simulink model "DCDC3_ZCL"  (R2024a)
settings: Solver=FixedStepDiscrete  StartTime=0.0  StopTime=Tsim_outLoop  FixedStep=Tsw  RelTol=1e-3
undefined symbols (not defined in the file): deadtimesw, ILmax, kaw_i, kaw_v, ki_i, ki_v, kp_i, kp_v, Rload, Tstep, Tsw, VinNom, VLlim, VoutNom, zden_aaf, zden_Integrator, zden_plant_i, zden_plant_v, znum_aaf, znum_Integrator, znum_plant_i, znum_plant_v
libraries: simulink x10, spsTriangleGeneratorLib x6
settings Model: Creator=nicholas  LastModifiedBy=nicholas
settings RTWCC: GPUComputeCapability=3.5

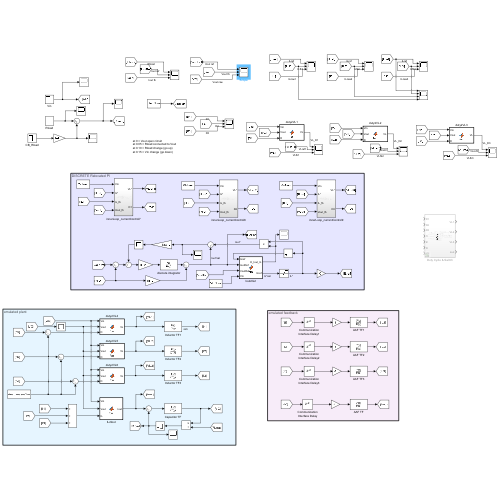
[thumbnail: Simulink's stored preview of the top-level diagram]
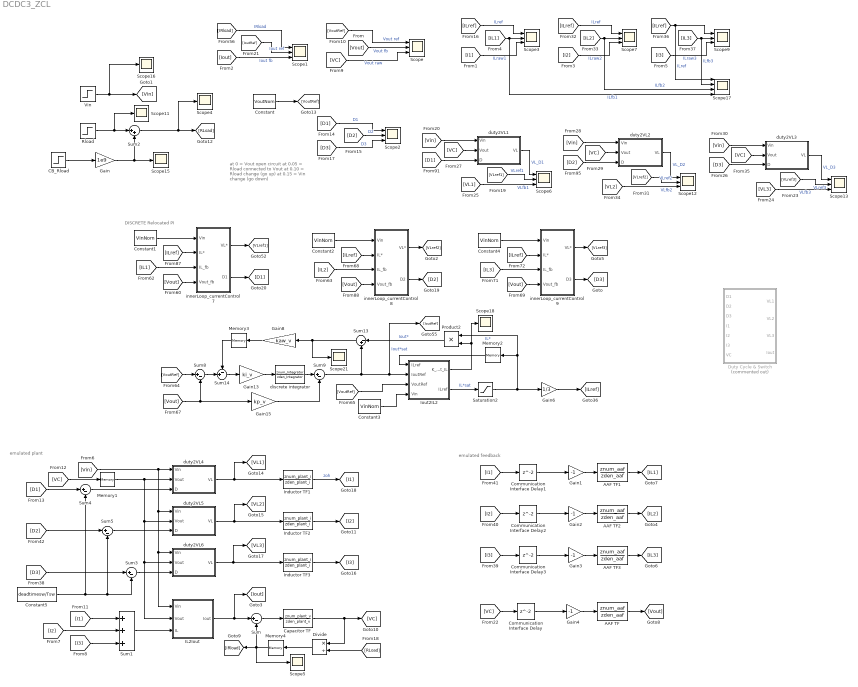
== system DCDC3_ZCL ==
  note: emulated plant
  note: emulated feedback
  note: DISCRETE Relocated PI
  note: at 0 = Vout open circuit
      | at 0.05 = Rload connected to Vout
      | at 0.10 = Rload change (go up)
      | at 0.15 = Vin change (go down)
  AAF TF{,1..3} (4 alike) : DiscreteTransferFcn  Numerator=znum_aaf  Denominator=zden_aaf
  CB_Rload : Step  Time=0.05  Before=1  After=0  SampleTime=0
  Capacitor TF : DiscreteTransferFcn  Numerator=znum_plant_v  Denominator=zden_plant_v
  Communication Interface Delay{,1..3} (4 alike) : Delay
  Constant : Constant  Value=VoutNom
  Constant{1..4} (4 alike) : Constant  Value=VinNom
  Constant5 : Constant  Value=deadtimesw/Tsw
  Divide : Product  Inputs=*/
  Duty Cycle & Switch : Subsystem  Commented=on
  Gain : Gain  Gain=1e9
  Gain{1..4} (4 alike) : Gain  Gain=-1
  Gain13 : Gain  Gain=ki_v
  Gain15 : Gain  Gain=kp_v
  Gain6 : Gain  Gain=1/3
  Gain8 : Gain  Gain=kaw_v
  IL2Iout : MATLAB Function  TreatAsAtomicUnit=on
  Inductor TF1 : DiscreteTransferFcn  Numerator=znum_plant_i  Denominator=zden_plant_i
  Inductor TF2 : DiscreteTransferFcn  Numerator=znum_plant_i  Denominator=zden_plant_i
  Inductor TF3 : DiscreteTransferFcn  Numerator=znum_plant_i  Denominator=zden_plant_i
  Iout2IL2 : MATLAB Function  TreatAsAtomicUnit=on
  Memory{1..4} (4 alike) : Memory  InheritSampleTime=on
  Product2 : Product
  Rload : Step  Time=0.10  Before=Rload  After=Rload*2  SampleTime=0
  Saturation2 : Saturate  UpperLimit=ILmax  LowerLimit=-ILmax
  Scope{,1..3,6..7,9,12..13} (9 alike) : Scope  NumInputPorts=3
  Scope{4..5,11,15..16,18,21} (7 alike) : Scope
  Scope17 : Scope  NumInputPorts=4
  Sum{,3..5,8..9} (6 alike) : Sum  Inputs=|+-
  Sum1 : Sum  Inputs=+++
  Sum13 : Sum  Inputs=|-+
  Sum14 : Sum  Inputs=-+|
  Sum2 : Sum  Inputs=|++
  Vin : Step  Time=0.15  Before=VinNom  After=20  SampleTime=0
  discrete integrator : DiscreteTransferFcn  Numerator=znum_Integrator  Denominator=zden_Integrator
  duty2VL1 : MATLAB Function  TreatAsAtomicUnit=on
  duty2VL2 : MATLAB Function  TreatAsAtomicUnit=on
  duty2VL3 : MATLAB Function  TreatAsAtomicUnit=on
  duty2VL4 : MATLAB Function  TreatAsAtomicUnit=on
  duty2VL5 : MATLAB Function  TreatAsAtomicUnit=on
  duty2VL6 : MATLAB Function  TreatAsAtomicUnit=on
  innerLoop_currentControl7 : Subsystem
  innerLoop_currentControl8 : Subsystem
  innerLoop_currentControl9 : Subsystem
  wires:
  [Iout] -> Scope1/3  "Iout fb"
  [Vout] -> Scope/2  "Vout fb"
  [IL1] -> Scope17/4, Scope3/2  "ILfb1"
  [ILref] -> Scope3/1  "ILref"
  [VoutRef] -> Scope/1  "Vout ref"
  [IoutRef] -> Scope1/2  "Iout ref"
  Constant/1 -> [VoutRef]
  [IL2] -> Scope7/2, Scope17/3  "ILfb2"
  [ILref] -> Scope7/1  "ILref"
  [IL3] -> Scope17/2, Scope9/2  "ILfb3"
  [ILref] -> Scope17/1, Scope9/1  "ILref"
  [IRload] -> Scope1/1  "IRload"
  [I1] -> Scope3/3  "ILraw1"
  [I2] -> Scope7/3  "ILraw2"
  [I3] -> Scope9/3  "ILraw3"
  Saturation2/1 -> Product2/1, Memory2/1, Gain6/1  "IL*"
  [IL1] -> innerLoop_currentControl7/3(IL_fb)
  [Vout] -> innerLoop_currentControl8/4(Vout_fb)
  Constant4/1 -> innerLoop_currentControl9/1(Vin)
  Gain13/1 -> discrete integrator/1
  [VoutRef] -> Sum8/1
  [Vout] -> innerLoop_currentControl7/4(Vout_fb)
  Constant1/1 -> innerLoop_currentControl7/1(Vin)
  discrete integrator/1 -> Sum9/1
  Constant3/1 -> Iout2IL2/4(Vin)
  [ILref] -> innerLoop_currentControl8/2(IL*)
  Product2/1 -> Sum13/1  "Iout*"
  Iout2IL2/2(ILref) -> Saturation2/1  "IL*sat"
  [IL3] -> innerLoop_currentControl9/3(IL_fb)
  [IL2] -> innerLoop_currentControl8/3(IL_fb)
  [VoutRef] -> Iout2IL2/3(VoutRef)
  Gain8/1 -> Memory3/1
  Gain6/1 -> [ILref]
  [Vout] -> Gain15/1, Sum8/2
  Sum9/1 -> Sum13/2, Iout2IL2/2(IoutRef), [IoutRef]  "Iout*sat"
  [ILref] -> innerLoop_currentControl7/2(IL*)
  Sum8/1 -> Sum14/2
  Sum14/1 -> Gain13/1
  Constant2/1 -> innerLoop_currentControl8/1(Vin)
  [ILref] -> innerLoop_currentControl9/2(IL*)
  [Vout] -> innerLoop_currentControl9/4(Vout_fb)
  Sum13/1 -> Scope21/1, Gain8/1
  Gain15/1 -> Sum9/2
  Inductor TF2/1 -> [I2]
  Inductor TF3/1 -> [I3]
  Capacitor TF/1 -> [VC], Divide/1
  Divide/1 -> Memory4/1
  innerLoop_currentControl9/2(D3) -> [D3]
  innerLoop_currentControl8/2(D2) -> [D2]
  innerLoop_currentControl7/2(D1) -> [D1]
  [I1] -> Sum1/1
  [I2] -> Sum1/2
  [I3] -> Sum1/3
  innerLoop_currentControl7/1(VL*) -> [VLref1]
  innerLoop_currentControl8/1(VL*) -> [VLref2]
  innerLoop_currentControl9/1(VL*) -> [VLref3]
  Communication Interface Delay/1 -> Gain4/1
  [D3] -> Scope2/3  "D3"
  [D1] -> Scope2/1  "D1"
  [D2] -> Scope2/2  "D2"
  [VC] -> Scope/3  "Vout raw"
  Vin/1 -> Scope16/1, [Vin]
  CB_Rload/1 -> Gain/1
  Sum/1 -> Capacitor TF/1
  Rload/1 -> Scope11/1, Sum2/1
  duty2VL3/1(VL) -> Scope13/1  "VL_D3"
  duty2VL2/1(VL) -> Scope12/1  "VL_D2"
  duty2VL1/1(VL) -> Scope6/1  "VL_D1"
  [VLref3] -> Scope13/2  "VLref3"
  [VLref2] -> Scope12/2  "VLref2"
  [VLref1] -> Scope6/2  "VLref1"
  [VL3] -> Scope13/3  "VLfb3"
  [VL1] -> Scope6/3  "VLfb1"
  [VL2] -> Scope12/3  "VLfb2"
  [D1] -> duty2VL1/3(D)
  [Vin] -> duty2VL1/1(Vin)
  [VC] -> duty2VL1/2(Vout)
  [D2] -> duty2VL2/3(D)
  [VC] -> duty2VL2/2(Vout)
  [Vin] -> duty2VL2/1(Vin)
  [D3] -> duty2VL3/3(D)
  [VC] -> duty2VL3/2(Vout)
  [Vin] -> duty2VL3/1(Vin)
  [Vin] -> duty2VL4/1(Vin), duty2VL6/1(Vin), IL2Iout/1(Vin), duty2VL5/1(Vin)
  duty2VL6/1(VL) -> [VL3], Inductor TF3/1
  duty2VL5/1(VL) -> [VL2], Inductor TF2/1
  [RLoad] -> Divide/2
  Gain/1 -> Sum2/2, Scope15/1
  Sum2/1 -> Scope4/1, [RLoad]
  [VC] -> Memory1/1
  Communication Interface Delay1/1 -> Gain1/1
  Inductor TF1/1 -> [I1]  "zoh"
  Communication Interface Delay2/1 -> Gain2/1
  Communication Interface Delay3/1 -> Gain3/1
  AAF TF3/1 -> [IL3]
  Gain3/1 -> AAF TF3/1
  AAF TF2/1 -> [IL2]
  Gain2/1 -> AAF TF2/1
  Gain1/1 -> AAF TF1/1
  AAF TF1/1 -> [IL1]
  AAF TF/1 -> [Vout]
  Gain4/1 -> AAF TF/1
  Sum1/1 -> IL2Iout/3(IL)
  IL2Iout/1(Iout) -> [Iout], Sum/1
  [VC] -> Communication Interface Delay/1
  [I3] -> Communication Interface Delay3/1
  [I2] -> Communication Interface Delay2/1
  [I1] -> Communication Interface Delay1/1
  duty2VL4/1(VL) -> [VL1], Inductor TF1/1
  Memory1/1 -> IL2Iout/2(Vout), duty2VL6/2(Vout), duty2VL5/2(Vout), duty2VL4/2(Vout)
  Iout2IL2/1(K_Iout_IL) -> Product2/2, Scope18/1
  Memory4/1 -> Scope5/1, [IRload], Sum/2
  Memory2/1 -> Iout2IL2/1("ILref ")
  Memory3/1 -> Sum14/1
  Constant5/1 -> Sum5/2, Sum3/2, Sum4/2
  Sum3/1 -> duty2VL6/3(D)
  [D3] -> Sum3/1
  [D2] -> Sum5/1
  [D1] -> Sum4/1
  Sum4/1 -> duty2VL4/3(D)
  Sum5/1 -> duty2VL5/3(D)

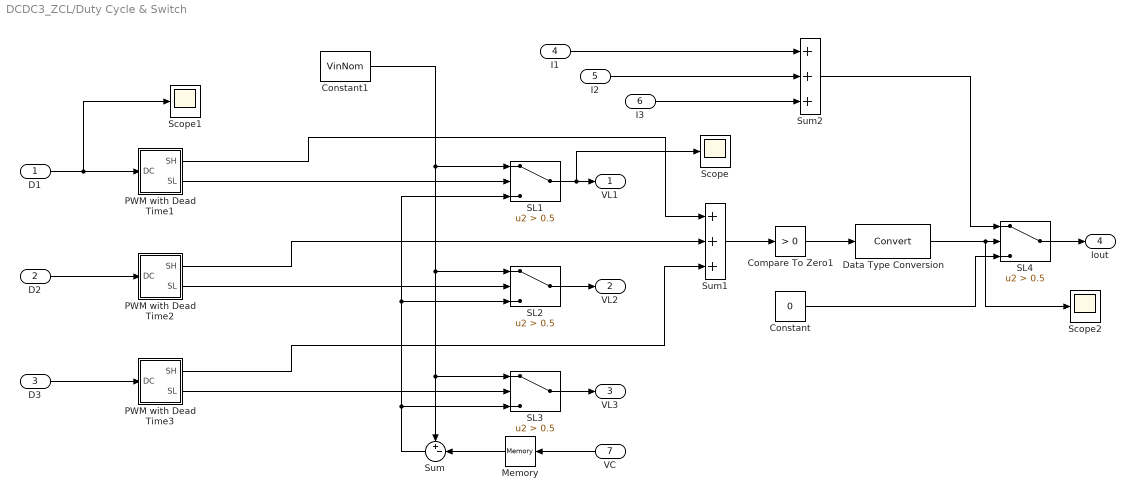
== system DCDC3_ZCL/Duty Cycle & Switch ==
  D1 : Inport
  D2 : Inport  Port=2
  D3 : Inport  Port=3
  I1 : Inport  Port=4
  I2 : Inport  Port=5
  I3 : Inport  Port=6
  VC : Inport  Port=7
  Compare To Zero1 : simulink/Logic and Bit Operations/Compare To Zero  relop=>  OutDataTypeStr=boolean
  Constant : Constant  Value=0
  Constant1 : Constant  Value=VinNom
  Data Type Conversion : DataTypeConversion  SaturateOnIntegerOverflow=off  RndMeth=Floor
  Memory : Memory
  PWM with Dead Time1 : Subsystem
  PWM with Dead Time2 : Subsystem
  PWM with Dead Time3 : Subsystem
  SL{1..4} (4 alike) : Switch  Criteria=u2 > Threshold  Threshold=0.5  SaturateOnIntegerOverflow=off  InputSameDT=off
  Scope : Scope
  Scope1 : Scope
  Scope2 : Scope
  Sum : Sum  Inputs=+-|
  Sum1 : Sum  Inputs=+++
  Sum2 : Sum  Inputs=+++
  VL1 : Outport
  VL2 : Outport  Port=2
  VL3 : Outport  Port=3
  Iout : Outport  Port=4
  wires:
  D1/1 -> Scope1/1, PWM with Dead Time1/1(DC)
  D2/1 -> PWM with Dead Time2/1(DC)
  PWM with Dead Time2/2(SL) -> SL2/2
  PWM with Dead Time3/2(SL) -> SL3/2
  Constant1/1 -> SL1/1, SL2/1, SL3/1, Sum/1
  PWM with Dead Time1/2(SL) -> SL1/2
  PWM with Dead Time3/1(SH) -> Sum1/3
  PWM with Dead Time2/1(SH) -> Sum1/2
  PWM with Dead Time1/1(SH) -> Sum1/1
  SL1/1 -> Scope/1, VL1/1
  SL2/1 -> VL2/1
  SL3/1 -> VL3/1
  Sum/1 -> SL1/3, SL2/3, SL3/3
  Sum1/1 -> Compare To Zero1/1
  Compare To Zero1/1 -> Data Type Conversion/1
  Sum2/1 -> SL4/1
  Constant/1 -> SL4/3
  SL4/1 -> Iout/1
  I1/1 -> Sum2/1
  I2/1 -> Sum2/2
  I3/1 -> Sum2/3
  Data Type Conversion/1 -> Scope2/1, SL4/2
  D3/1 -> PWM with Dead Time3/1(DC)
  VC/1 -> Memory/1
  Memory/1 -> Sum/2

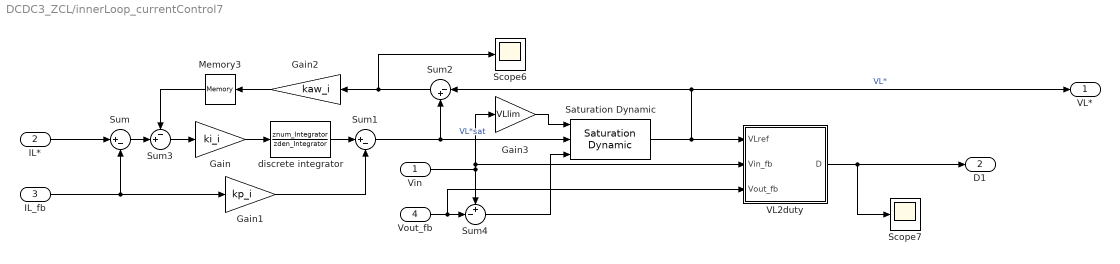
== system DCDC3_ZCL/innerLoop_currentControl7 ==
  Vin : Inport
  IL* : Inport  Port=2
  IL_fb : Inport  Port=3
  Vout_fb : Inport  Port=4
  Gain : Gain  Gain=ki_i
  Gain1 : Gain  Gain=kp_i
  Gain2 : Gain  Gain=kaw_i
  Gain3 : Gain  Gain=VLlim
  Memory3 : Memory  InheritSampleTime=on
  Saturation Dynamic : simulink/Discontinuities/Saturation Dynamic  OutMin=[]  OutMax=[]  OutDataTypeStr=Inherit: Same as second input  OutDataType=fixdt(1, 16)  OutScaling=2^-10  DoSatur=off
  Scope6 : Scope
  Scope7 : Scope
  Sum : Sum  Inputs=|+-
  Sum1 : Sum  Inputs=|+-
  Sum2 : Sum  Inputs=|-+
  Sum3 : Sum  Inputs=-+|
  Sum4 : Sum  Inputs=+-|
  VL2duty : MATLAB Function  TreatAsAtomicUnit=on
  discrete integrator : DiscreteTransferFcn  Numerator=znum_Integrator  Denominator=zden_Integrator
  VL* : Outport
  D1 : Outport  Port=2
  wires:
  VL2duty/1(D) -> D1/1, Scope7/1
  Sum/1 -> Sum3/2
  Gain3/1 -> Saturation Dynamic/1
  Gain1/1 -> Sum1/2
  Sum3/1 -> Gain/1
  Gain/1 -> discrete integrator/1
  Gain2/1 -> Memory3/1
  Vin/1 -> VL2duty/2(Vin_fb), Gain3/1, Sum4/1
  Sum1/1 -> Saturation Dynamic/2, Sum2/2  "VL*sat"
  Sum4/1 -> Saturation Dynamic/3
  Sum2/1 -> Gain2/1, Scope6/1
  Saturation Dynamic/1 -> VL*/1, Sum2/1, VL2duty/1(VLref)  "VL*"
  IL_fb/1 -> Sum/2, Gain1/1
  Vout_fb/1 -> VL2duty/3(Vout_fb), Sum4/2
  discrete integrator/1 -> Sum1/1
  IL*/1 -> Sum/1
  Memory3/1 -> Sum3/1

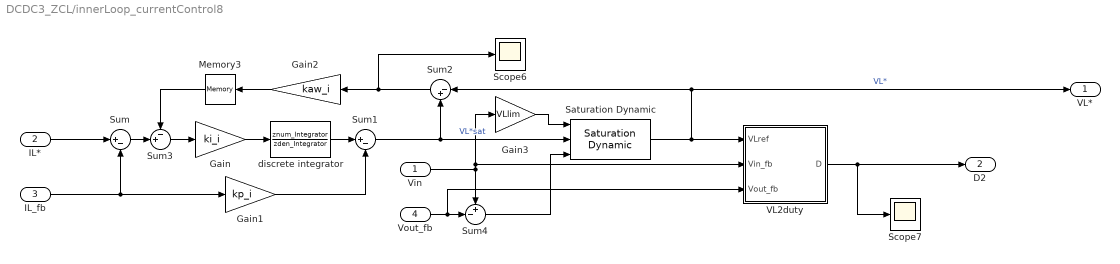
== system DCDC3_ZCL/innerLoop_currentControl8 ==
  Vin : Inport
  IL* : Inport  Port=2
  IL_fb : Inport  Port=3
  Vout_fb : Inport  Port=4
  Gain : Gain  Gain=ki_i
  Gain1 : Gain  Gain=kp_i
  Gain2 : Gain  Gain=kaw_i
  Gain3 : Gain  Gain=VLlim
  Memory3 : Memory  InheritSampleTime=on
  Saturation Dynamic : simulink/Discontinuities/Saturation Dynamic  OutMin=[]  OutMax=[]  OutDataTypeStr=Inherit: Same as second input  OutDataType=fixdt(1, 16)  OutScaling=2^-10  DoSatur=off
  Scope6 : Scope
  Scope7 : Scope
  Sum : Sum  Inputs=|+-
  Sum1 : Sum  Inputs=|+-
  Sum2 : Sum  Inputs=|-+
  Sum3 : Sum  Inputs=-+|
  Sum4 : Sum  Inputs=+-|
  VL2duty : MATLAB Function  TreatAsAtomicUnit=on
  discrete integrator : DiscreteTransferFcn  Numerator=znum_Integrator  Denominator=zden_Integrator
  VL* : Outport
  D2 : Outport  Port=2
  wires:
  Sum/1 -> Sum3/2
  Gain3/1 -> Saturation Dynamic/1
  Gain1/1 -> Sum1/2
  Sum3/1 -> Gain/1
  Gain/1 -> discrete integrator/1
  Gain2/1 -> Memory3/1
  Vin/1 -> VL2duty/2(Vin_fb), Gain3/1, Sum4/1
  Sum1/1 -> Saturation Dynamic/2, Sum2/2  "VL*sat"
  Sum4/1 -> Saturation Dynamic/3
  Sum2/1 -> Gain2/1, Scope6/1
  Saturation Dynamic/1 -> VL*/1, Sum2/1, VL2duty/1(VLref)  "VL*"
  Vout_fb/1 -> VL2duty/3(Vout_fb), Sum4/2
  discrete integrator/1 -> Sum1/1
  IL*/1 -> Sum/1
  VL2duty/1(D) -> D2/1, Scope7/1
  IL_fb/1 -> Sum/2, Gain1/1
  Memory3/1 -> Sum3/1

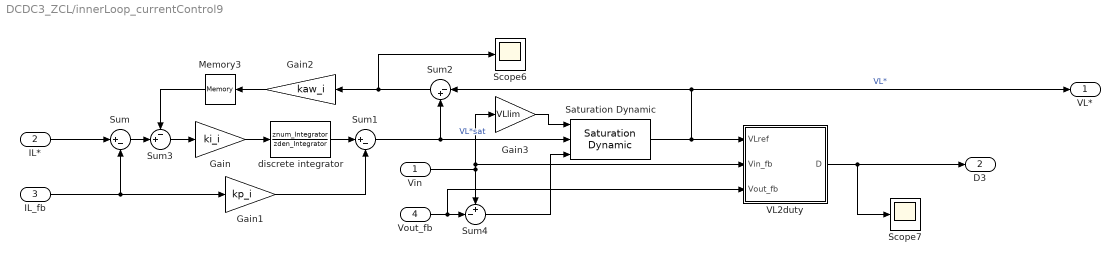
== system DCDC3_ZCL/innerLoop_currentControl9 ==
  Vin : Inport
  IL* : Inport  Port=2
  IL_fb : Inport  Port=3
  Vout_fb : Inport  Port=4
  Gain : Gain  Gain=ki_i
  Gain1 : Gain  Gain=kp_i
  Gain2 : Gain  Gain=kaw_i
  Gain3 : Gain  Gain=VLlim
  Memory3 : Memory  InheritSampleTime=on
  Saturation Dynamic : simulink/Discontinuities/Saturation Dynamic  OutMin=[]  OutMax=[]  OutDataTypeStr=Inherit: Same as second input  OutDataType=fixdt(1, 16)  OutScaling=2^-10  DoSatur=off
  Scope6 : Scope
  Scope7 : Scope
  Sum : Sum  Inputs=|+-
  Sum1 : Sum  Inputs=|+-
  Sum2 : Sum  Inputs=|-+
  Sum3 : Sum  Inputs=-+|
  Sum4 : Sum  Inputs=+-|
  VL2duty : MATLAB Function  TreatAsAtomicUnit=on
  discrete integrator : DiscreteTransferFcn  Numerator=znum_Integrator  Denominator=zden_Integrator
  VL* : Outport
  D3 : Outport  Port=2
  wires:
  Sum/1 -> Sum3/2
  Gain3/1 -> Saturation Dynamic/1
  Gain1/1 -> Sum1/2
  Sum3/1 -> Gain/1
  Gain/1 -> discrete integrator/1
  Gain2/1 -> Memory3/1
  Vin/1 -> VL2duty/2(Vin_fb), Gain3/1, Sum4/1
  Sum1/1 -> Saturation Dynamic/2, Sum2/2  "VL*sat"
  Sum4/1 -> Saturation Dynamic/3
  Sum2/1 -> Gain2/1, Scope6/1
  Saturation Dynamic/1 -> VL*/1, Sum2/1, VL2duty/1(VLref)  "VL*"
  IL_fb/1 -> Sum/2, Gain1/1
  Vout_fb/1 -> VL2duty/3(Vout_fb), Sum4/2
  discrete integrator/1 -> Sum1/1
  IL*/1 -> Sum/1
  VL2duty/1(D) -> D3/1, Scope7/1
  Memory3/1 -> Sum3/1

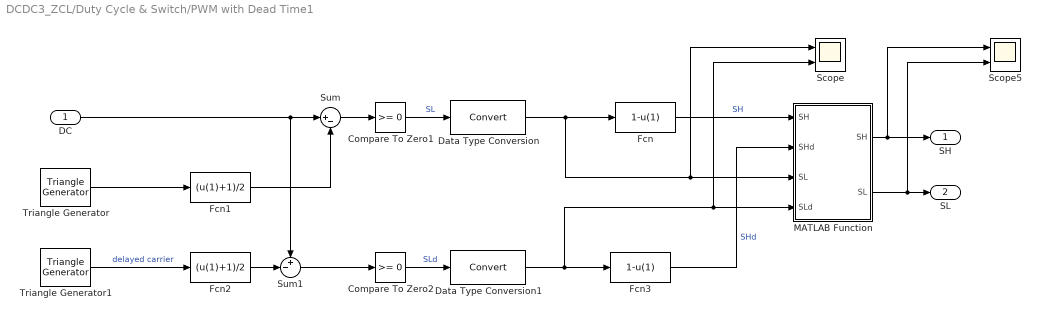
== system DCDC3_ZCL/Duty Cycle & Switch/PWM with Dead Time1 ==
  DC : Inport
  Compare To Zero1 : simulink/Logic and Bit Operations/Compare To Zero  relop=>=  OutDataTypeStr=boolean
  Compare To Zero2 : simulink/Logic and Bit Operations/Compare To Zero  relop=>=  OutDataTypeStr=boolean
  Data Type Conversion : DataTypeConversion  SaturateOnIntegerOverflow=off  RndMeth=Floor
  Data Type Conversion1 : DataTypeConversion  SaturateOnIntegerOverflow=off  RndMeth=Floor
  Fcn : Fcn  Expr=1-u(1)
  Fcn1 : Fcn  Expr=(u(1)+1)/2
  Fcn2 : Fcn  Expr=(u(1)+1)/2
  Fcn3 : Fcn  Expr=1-u(1)
  MATLAB Function : MATLAB Function  TreatAsAtomicUnit=on
  Scope : Scope  NumInputPorts=2
  Scope5 : Scope  NumInputPorts=2
  Sum : Sum  Inputs=|+-
  Sum1 : Sum  Inputs=+-|
  Triangle Generator : spsTriangleGeneratorLib/Triangle Generator  Freq=fsw  Phase=0  Ts=Tstep
  Triangle Generator1 : spsTriangleGeneratorLib/Triangle Generator  Freq=fsw  Phase=-(deadtimesw/Tsw)*360  Ts=Tstep
  SH : Outport
  SL : Outport  Port=2
  wires:
  Compare To Zero1/1 -> Data Type Conversion/1  "SL"
  Fcn/1 -> MATLAB Function/1("SH ")  "SH"
  MATLAB Function/2(SL) -> SL/1, Scope5/2
  MATLAB Function/1(SH) -> SH/1, Scope5/1
  DC/1 -> Sum1/1, Sum/1
  Triangle Generator/1 -> Fcn1/1
  Sum/1 -> Compare To Zero1/1
  Fcn1/1 -> Sum/2
  Triangle Generator1/1 -> Fcn2/1  "delayed carrier"
  Sum1/1 -> Compare To Zero2/1
  Fcn2/1 -> Sum1/2
  Compare To Zero2/1 -> Data Type Conversion1/1  "SLd"
  Fcn3/1 -> MATLAB Function/2(SHd)  "SHd"
  Data Type Conversion/1 -> Fcn/1, Scope/1, MATLAB Function/3("SL ")
  Data Type Conversion1/1 -> Fcn3/1, Scope/2, MATLAB Function/4(SLd)

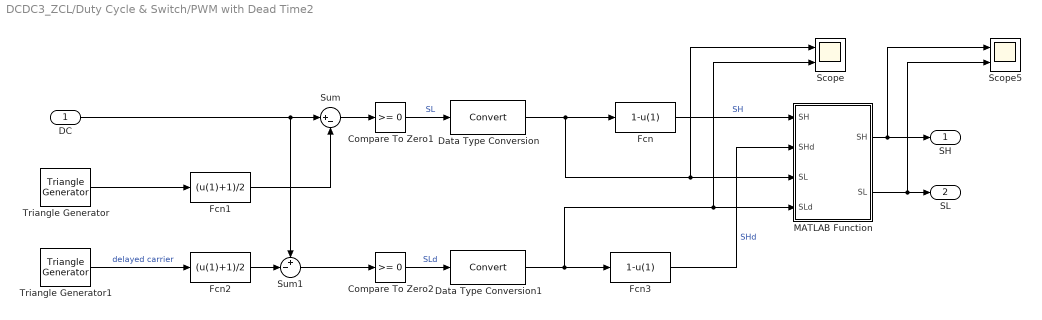
== system DCDC3_ZCL/Duty Cycle & Switch/PWM with Dead Time2 ==
  DC : Inport
  Compare To Zero1 : simulink/Logic and Bit Operations/Compare To Zero  relop=>=  OutDataTypeStr=boolean
  Compare To Zero2 : simulink/Logic and Bit Operations/Compare To Zero  relop=>=  OutDataTypeStr=boolean
  Data Type Conversion : DataTypeConversion  SaturateOnIntegerOverflow=off  RndMeth=Floor
  Data Type Conversion1 : DataTypeConversion  SaturateOnIntegerOverflow=off  RndMeth=Floor
  Fcn : Fcn  Expr=1-u(1)
  Fcn1 : Fcn  Expr=(u(1)+1)/2
  Fcn2 : Fcn  Expr=(u(1)+1)/2
  Fcn3 : Fcn  Expr=1-u(1)
  MATLAB Function : MATLAB Function  TreatAsAtomicUnit=on
  Scope : Scope  NumInputPorts=2
  Scope5 : Scope  NumInputPorts=2
  Sum : Sum  Inputs=|+-
  Sum1 : Sum  Inputs=+-|
  Triangle Generator : spsTriangleGeneratorLib/Triangle Generator  Freq=fsw  Phase=120  Ts=Tstep
  Triangle Generator1 : spsTriangleGeneratorLib/Triangle Generator  Freq=fsw  Phase=120-(deadtimesw/Tsw)*360  Ts=Tstep
  SH : Outport
  SL : Outport  Port=2
  wires:
  Compare To Zero1/1 -> Data Type Conversion/1  "SL"
  Fcn/1 -> MATLAB Function/1("SH ")  "SH"
  MATLAB Function/2(SL) -> SL/1, Scope5/2
  MATLAB Function/1(SH) -> SH/1, Scope5/1
  DC/1 -> Sum1/1, Sum/1
  Triangle Generator/1 -> Fcn1/1
  Sum/1 -> Compare To Zero1/1
  Fcn1/1 -> Sum/2
  Triangle Generator1/1 -> Fcn2/1  "delayed carrier"
  Sum1/1 -> Compare To Zero2/1
  Fcn2/1 -> Sum1/2
  Compare To Zero2/1 -> Data Type Conversion1/1  "SLd"
  Fcn3/1 -> MATLAB Function/2(SHd)  "SHd"
  Data Type Conversion/1 -> Fcn/1, Scope/1, MATLAB Function/3("SL ")
  Data Type Conversion1/1 -> Fcn3/1, Scope/2, MATLAB Function/4(SLd)

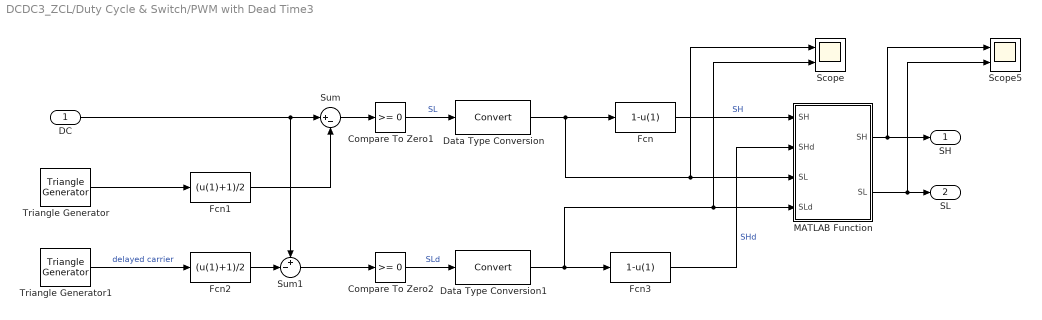
== system DCDC3_ZCL/Duty Cycle & Switch/PWM with Dead Time3 ==
  DC : Inport
  Compare To Zero1 : simulink/Logic and Bit Operations/Compare To Zero  relop=>=  OutDataTypeStr=boolean
  Compare To Zero2 : simulink/Logic and Bit Operations/Compare To Zero  relop=>=  OutDataTypeStr=boolean
  Data Type Conversion : DataTypeConversion  SaturateOnIntegerOverflow=off  RndMeth=Floor
  Data Type Conversion1 : DataTypeConversion  SaturateOnIntegerOverflow=off  RndMeth=Floor
  Fcn : Fcn  Expr=1-u(1)
  Fcn1 : Fcn  Expr=(u(1)+1)/2
  Fcn2 : Fcn  Expr=(u(1)+1)/2
  Fcn3 : Fcn  Expr=1-u(1)
  MATLAB Function : MATLAB Function  TreatAsAtomicUnit=on
  Scope : Scope  NumInputPorts=2
  Scope5 : Scope  NumInputPorts=2
  Sum : Sum  Inputs=|+-
  Sum1 : Sum  Inputs=+-|
  Triangle Generator : spsTriangleGeneratorLib/Triangle Generator  Freq=fsw  Phase=240  Ts=Tstep
  Triangle Generator1 : spsTriangleGeneratorLib/Triangle Generator  Freq=fsw  Phase=240-(deadtimesw/Tsw)*360  Ts=Tstep
  SH : Outport
  SL : Outport  Port=2
  wires:
  Compare To Zero1/1 -> Data Type Conversion/1  "SL"
  Fcn/1 -> MATLAB Function/1("SH ")  "SH"
  MATLAB Function/2(SL) -> SL/1, Scope5/2
  MATLAB Function/1(SH) -> SH/1, Scope5/1
  DC/1 -> Sum1/1, Sum/1
  Triangle Generator/1 -> Fcn1/1
  Sum/1 -> Compare To Zero1/1
  Fcn1/1 -> Sum/2
  Triangle Generator1/1 -> Fcn2/1  "delayed carrier"
  Sum1/1 -> Compare To Zero2/1
  Fcn2/1 -> Sum1/2
  Compare To Zero2/1 -> Data Type Conversion1/1  "SLd"
  Fcn3/1 -> MATLAB Function/2(SHd)  "SHd"
  Data Type Conversion/1 -> Fcn/1, Scope/1, MATLAB Function/3("SL ")
  Data Type Conversion1/1 -> Fcn3/1, Scope/2, MATLAB Function/4(SLd)

== matlab function DCDC3_ZCL/duty2VL6 ==
  data: Vin input; Vout input; D input; VL output
function VL = fcn(Vin,Vout,D)

VL = min((D-1)*Vout + Vin, Vin);

== matlab function DCDC3_ZCL/IL2Iout ==
  data: Vin input; Vout input; Iout output; IL input; RserL parameter
function Iout = fcn(Vin,Vout,IL,RserL)

if Vout < Vin
    Vout = Vin;
end
K_Iout_IL = (Vin - RserL*IL) / Vout;
Iout = IL*K_Iout_IL;

== matlab function DCDC3_ZCL/innerLoop_currentControl7/VL2duty ==
  data: VLref input; D output; Vin_fb input; Vout_fb input
function D = fcn(VLref,Vin_fb,Vout_fb)
% Vout = Vin * 1/(1-D) where Vin = Vs-VL
% Vout/(Vs - VL) = 1/(1-D)
D = min([1 max([0 (1 + (VLref - Vin_fb)/Vout_fb)])]);

== matlab function DCDC3_ZCL/innerLoop_currentControl8/VL2duty ==
  data: VLref input; D output; Vin_fb input; Vout_fb input
function D = fcn(VLref,Vin_fb,Vout_fb)
% Vout = Vin * 1/(1-D) where Vin = Vs-VL
% Vout/(Vs - VL) = 1/(1-D)
D = min([1 max([0 (1 + (VLref - Vin_fb)/Vout_fb)])]);

== matlab function DCDC3_ZCL/innerLoop_currentControl9/VL2duty ==
  data: VLref input; D output; Vin_fb input; Vout_fb input
function D = fcn(VLref,Vin_fb,Vout_fb)
% Vout = Vin * 1/(1-D) where Vin = Vs-VL
% Vout/(Vs - VL) = 1/(1-D)
D = min([1 max([0 (1 + (VLref - Vin_fb)/Vout_fb)])]);

== matlab function DCDC3_ZCL/Duty Cycle & Switch/PWM with Dead Time1/MATLAB Function ==
  data: SH input; SHd input; SH output; SL output; SL input; SLd input
function [SH,SL] = fcn(SH,SHd,SL,SLd)

if SHd + SH > 1
    SH = 1;
else
    SH = 0;
end

if SLd + SL > 1
    SL = 1;
else
    SL = 0;
end

== matlab function DCDC3_ZCL/Duty Cycle & Switch/PWM with Dead Time2/MATLAB Function ==
  data: SH input; SHd input; SH output; SL output; SL input; SLd input
function [SH,SL] = fcn(SH,SHd,SL,SLd)

if SHd + SH > 1
    SH = 1;
else
    SH = 0;
end

if SLd + SL > 1
    SL = 1;
else
    SL = 0;
end

== matlab function DCDC3_ZCL/Duty Cycle & Switch/PWM with Dead Time3/MATLAB Function ==
  data: SH input; SHd input; SH output; SL output; SL input; SLd input
function [SH,SL] = fcn(SH,SHd,SL,SLd)

if SHd + SH > 1
    SH = 1;
else
    SH = 0;
end

if SLd + SL > 1
    SL = 1;
else
    SL = 0;
end

== matlab function DCDC3_ZCL/duty2VL1 ==
  data: Vin input; Vout input; D input; VL output
function VL = fcn(Vin,Vout,D)

VL = (D-1)*Vout + Vin;

== matlab function DCDC3_ZCL/duty2VL2 ==
  data: Vin input; Vout input; D input; VL output
function VL = fcn(Vin,Vout,D)

VL = (D-1)*Vout + Vin;

== matlab function DCDC3_ZCL/duty2VL3 ==
  data: Vin input; Vout input; D input; VL output
function VL = fcn(Vin,Vout,D)

VL = (D-1)*Vout + Vin;

== matlab function DCDC3_ZCL/duty2VL4 ==
  data: Vin input; Vout input; D input; VL output
function VL = fcn(Vin,Vout,D)

VL = min((D-1)*Vout + Vin, Vin);

== matlab function DCDC3_ZCL/Iout2IL2 ==
  data: K_Iout_IL output; ILref input; IoutRef input; VoutRef input; Vin input; ILref output; RserL parameter
function [K_Iout_IL,ILref] = fcn(ILref,IoutRef,VoutRef,Vin,RserL)

if VoutRef < Vin
    VoutRef = Vin;
end
K_Iout_IL = (Vin - RserL*ILref) / VoutRef;
ILref = IoutRef / K_Iout_IL;

== matlab function DCDC3_ZCL/duty2VL5 ==
  data: Vin input; Vout input; D input; VL output
function VL = fcn(Vin,Vout,D)

VL = min((D-1)*Vout + Vin, Vin);
